simulink model "two_level_seriesparallel_spwm"  (R2016a)
settings: Solver=VariableStepAuto  StartTime=0.0  StopTime=stop_time  RelTol=1e-3
values from neighbouring files (symbols this model uses):
  DC_Voltage_Source = 540    [spectrumanalysis.m]
  DCLINK1_Cap = 100e-6    (= 0.0001)    [spectrumanalysis.m]
  DCLINK2_Cap = 100e-6    (= 0.0001)    [spectrumanalysis.m]
  interleaving_angle = 180    [spectrumanalysis.m]
  Load_Inductive_Power = 4116    [spectrumanalysis.m]
  Load_Real_Power = 8500    [spectrumanalysis.m]
  ma = 1    [spectrumanalysis.m]
  ref_frequency = 2*pi*50    (= 314.159265359)    [spectrumanalysis.m]
  Sampling_time = 1/(20*sw_frequency)    (= 2.43902439024e-05)    [spectrumanalysis.m]
libraries: powerlib x65, powerlib_meascontrol x12, simulink x12
settings Model: Creator=hakan  LastModifiedBy=hakan
settings DataIOCC: LimitDataPoints=on
settings DebuggingCC: MaxConsecutiveZCsMsg=none  AllowSymbolicDim=off
settings ModelReferenceCC: PropagateSignalLabelsOutOfModel=off
settings GRTTargetCC: GeneratePreprocessorConditionals=Use local settings

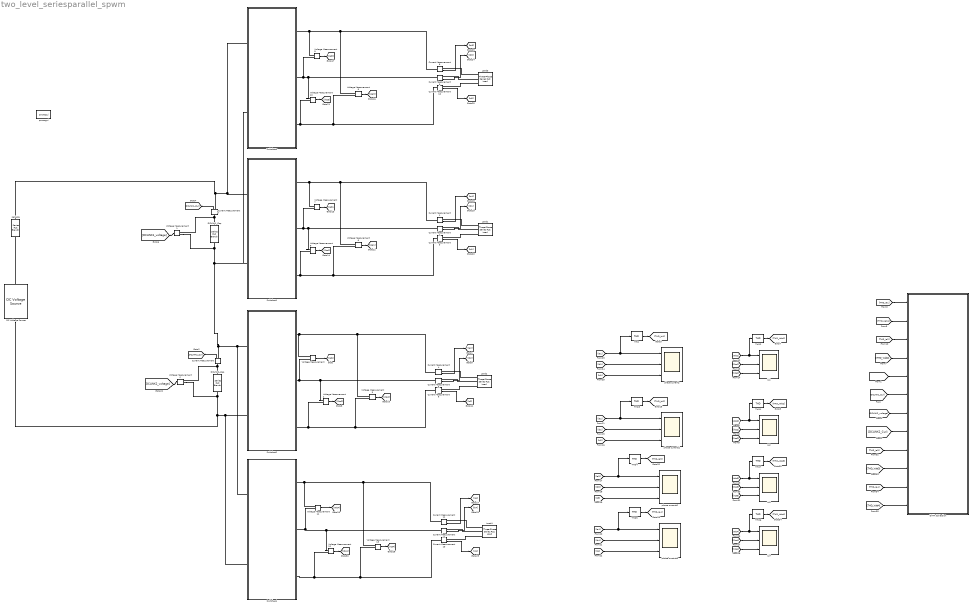
== system two_level_seriesparallel_spwm ==
  Current Measurement{,1..13} (14 alike) : powerlib/Measurements/Current Measurement  PhasorSimulation=off  OutputType=Complex  PSBequivalent=0
  DATA Collection : Subsystem
  DC Voltage Source : powerlib/Electrical Sources/DC Voltage Source  Amplitude=DC_Voltage_Source  Measurements=None
  DCLINK1_Cap : powerlib/Elements/Series RLC Branch  LConnTagsString=__new0  RConnTagsString=__new0  BranchType=C  Resistance=1  Inductance=1e-3  SetiL0=off  InitialCurrent=0  Capacitance=DCLINK1_Cap  Setx0=off  InitialVoltage=0  Measurements=None
  DCLINK2_Cap : powerlib/Elements/Series RLC Branch  LConnTagsString=__new0  RConnTagsString=__new0  BranchType=C  Resistance=1  Inductance=1e-3  SetiL0=off  InitialCurrent=0  Capacitance=DCLINK2_Cap  Setx0=off  InitialVoltage=0  Measurements=None
  LL{1..4} (4 alike) : Scope  NumInputPorts=3
  Load{1..4} (4 alike) : powerlib/Elements/Three-Phase Series RLC Load  LConnTagsString=A|B|C  Configuration=Y (floating)  NominalVoltage=1000  Vabc=[1e3 1e3 1e3]  Vabcp=[1e3 1e3 1e3]  NominalFrequency=Load_Nominal_Freq  UnbalancedPower=off  ActivePower=Load_Real_Power/4  InductivePower=Load_Inductive_Power/4  CapacitivePower=0  Pabc=[10e3 9e3 11e3]  QLabc=[100 90 110]  QCabc=[100 90 110]  Pabcp=[10e3 9e3 11e3]  QLabcp=[100 90 110]  QCabcp=[100 90 110]  Measurements=None  LoadType=constant Z
  Switches1 : Subsystem
  Switches2 : Subsystem
  Switches3 : Subsystem
  Switches4 : Subsystem
  THD{,1..7} (8 alike) : powerlib_meascontrol/Measurements/THD  Freq=50  Ts=0
  Voltage Measurement{,1..13} (14 alike) : powerlib/Measurements/Voltage Measurement  PhasorSimulation=off  OutputType=Complex  PSBequivalent=0
  phase currents{,1..3} (4 alike) : Scope  NumInputPorts=3
  powergui : powerlib/powergui  Priority=1  SimulationMode=Discrete  SolverType=Tustin/Backward Euler (TBE)  SampleTime=Sampling_time  frequency=60  SPID=off  DisableSnubberDevices=off  DisableRonSwitches=off  DisableVfSwitches=off  SwTol=0  DisplayEquations=off  Interpol=off  ExternalGateDelay=off  methode=off  Ts=10  FunctionMessages=off  echomessages=off  HookPort=off  EnableUseOfTLC=off  x0status=blocks  frequencyindice=0  Pbase=100e6  ErrMax=1e-4  Iterations=50  UnitsV=kV  UnitsW=MW  buscounter=0  RestoreLinks=warning  ResistiveCurrentMeasurement=off  Frange=[0:2:500]  Ylog=off  Xlog=on  ShowGrid=off  save=off  variable=ZData  structure=Phase_currents  ZoomFFT=off  StartTime=0.1  cycles=5  DisplayStyle=1  fundamental=50  FreqAxis=off  MaxFrequency=2000  frequencyindicesteady=1  RmsSteady=1  display=off
  seriesre : powerlib/Elements/Series RLC Branch  RequirementInfo={'linktype_rmi_matlab' 'C:\Users\hakan\Downloads\figuringout.m' '@737069.1' 'true' 'C' '' } %GIDa_c1573da4_5ff5_49fa_8615_7e57ae13da62  LConnTagsString=__new0  RConnTagsString=__new0  BranchType=R  Resistance=1  Inductance=1e-3  SetiL0=off  InitialCurrent=0  Capacitance=100e-6  Setx0=off  InitialVoltage=0  Measurements=Branch voltage and current
  wires:
  Current Measurement1/1 -> [Ia1]
  Current Measurement2/1 -> [Ib1]
  Current Measurement3/1 -> [Ic1]
  [Ib1] -> phase currents/2  "Ib"
  [Ia1] -> phase currents/1, THD/1  "Ia"
  [Ic1] -> phase currents/3  "Ic"
  [Vab1] -> THD2/1, LL1/1
  [Vbc1] -> LL1/2
  [Vca1] -> LL1/3
  THD/1 -> [THD_Ia1]
  [THD_Ia1] -> DATA Collection/1("THD_Ia1 ")
  THD2/1 -> [THD_Vab1]
  [THD_Vab2] -> DATA Collection/4(THD_Vab2)
  [THD_Vab1] -> DATA Collection/2(THD_Vab1)
  [DCLINK1_voltage] -> DATA Collection/5(DCLINK1_Voltage)
  [DCLINK1_Cur] -> DATA Collection/6(DCLINK1_Current)
  Current Measurement4/1 -> [Ia2]
  Current Measurement5/1 -> [Ib2]
  Current Measurement6/1 -> [Ic2]
  Voltage Measurement4/1 -> [DCLINK2_voltage]
  Current Measurement/1 -> [DCLINK2_Cur]
  Voltage Measurement1/1 -> [DCLINK1_voltage]
  Current Measurement7/1 -> [DCLINK1_Cur]
  [DCLINK2_voltage] -> DATA Collection/7(DCLINK2_Voltage)
  [DCLINK2_Cur] -> DATA Collection/8(DCLINK2_Current)
  Voltage Measurement/1 -> [Vab2]
  Voltage Measurement2/1 -> [Vbc2]
  Voltage Measurement3/1 -> [Vca2]
  Voltage Measurement6/1 -> [Vca1]
  Voltage Measurement7/1 -> [Vab1]
  Voltage Measurement8/1 -> [Vbc1]
  [Vab2] -> LL2/1, THD1/1
  [Vbc2] -> LL2/2
  [Vca2] -> LL2/3
  THD1/1 -> [THD_Vab2]
  [THD_Ia2] -> DATA Collection/3(THD_Ia2)
  [Ib2] -> phase currents1/2  "Ib"
  [Ia2] -> THD3/1, phase currents1/1  "Ia"
  [Ic2] -> phase currents1/3  "Ic"
  THD3/1 -> [THD_Ia2]
  Current Measurement8/1 -> [Ia3]
  Current Measurement9/1 -> [Ib3]
  Current Measurement10/1 -> [Ic3]
  Voltage Measurement5/1 -> [Vca3]
  Voltage Measurement9/1 -> [Vab3]
  Voltage Measurement10/1 -> [Vbc3]
  Current Measurement11/1 -> [Ia4]
  Current Measurement12/1 -> [Ib4]
  Current Measurement13/1 -> [Ic4]
  Voltage Measurement11/1 -> [Vab4]
  Voltage Measurement12/1 -> [Vbc4]
  Voltage Measurement13/1 -> [Vca4]
  [Ib3] -> phase currents2/2  "Ib"
  [Ia3] -> phase currents2/1, THD4/1  "Ia"
  [Ic3] -> phase currents2/3  "Ic"
  THD4/1 -> [THD_Ia3]
  [Ib4] -> phase currents3/2  "Ib"
  [Ia4] -> THD5/1, phase currents3/1  "Ia"
  [Ic4] -> phase currents3/3  "Ic"
  THD5/1 -> [THD_Ia4]
  [Vab4] -> THD6/1, LL4/1
  [Vbc4] -> LL4/2
  [Vca4] -> LL4/3
  THD6/1 -> [THD_Vab4]
  [Vab3] -> THD7/1, LL3/1
  [Vbc3] -> LL3/2
  [Vca3] -> LL3/3
  THD7/1 -> [THD_Vab3]
  [THD_Ia3] -> DATA Collection/9(THD_Ia3)
  [THD_Vab3] -> DATA Collection/10(THD_Vab3)
  [THD_Ia4] -> DATA Collection/11(THD_Ia4)
  [THD_Vab4] -> DATA Collection/12(THD_Vab4)
  connections:
  Load1/LConn1 -- Current Measurement1/RConn1
  Load1/LConn3 -- Current Measurement3/RConn1
  Load1/LConn2 -- Current Measurement2/RConn1
  Current Measurement1/LConn1 -- Voltage Measurement6/LConn2 -- Voltage Measurement7/LConn1 -- Switches1/RConn1
  Current Measurement2/LConn1 -- Voltage Measurement8/LConn1 -- Voltage Measurement7/LConn2 -- Switches1/RConn2
  Current Measurement3/LConn1 -- Voltage Measurement6/LConn1 -- Voltage Measurement8/LConn2 -- Switches1/RConn3
  Load2/LConn2 -- Current Measurement5/RConn1
  Load2/LConn3 -- Current Measurement6/RConn1
  Load2/LConn1 -- Current Measurement4/RConn1
  Current Measurement5/LConn1 -- Voltage Measurement2/LConn1 -- Voltage Measurement/LConn2 -- Switches2/RConn2
  Current Measurement4/LConn1 -- Voltage Measurement3/LConn2 -- Voltage Measurement/LConn1 -- Switches2/RConn1
  Current Measurement6/LConn1 -- Voltage Measurement3/LConn1 -- Voltage Measurement2/LConn2 -- Switches2/RConn3
  Voltage Measurement1/LConn2 -- Switches3/LConn2 -- Switches1/LConn2 -- Current Measurement/RConn1 -- Switches4/LConn1 -- Switches2/LConn1 -- DCLINK1_Cap/RConn1
  DC Voltage Source/LConn1 -- Voltage Measurement4/LConn2 -- DCLINK2_Cap/RConn1 -- Switches4/LConn2 -- Switches2/LConn2
  DC Voltage Source/RConn1 -- seriesre/RConn1
  seriesre/LConn1 -- Current Measurement7/RConn1 -- Switches3/LConn1 -- Switches1/LConn1
  DCLINK2_Cap/LConn1 -- Current Measurement/LConn1 -- Voltage Measurement4/LConn1
  DCLINK1_Cap/LConn1 -- Voltage Measurement1/LConn1 -- Current Measurement7/LConn1
  Current Measurement8/LConn1 -- Switches3/RConn1 -- Voltage Measurement9/LConn1 -- Voltage Measurement5/LConn2
  Current Measurement9/LConn1 -- Switches3/RConn2 -- Voltage Measurement9/LConn2 -- Voltage Measurement10/LConn1
  Current Measurement10/LConn1 -- Switches3/RConn3 -- Voltage Measurement10/LConn2 -- Voltage Measurement5/LConn1
  Load3/LConn3 -- Current Measurement10/RConn1
  Load3/LConn1 -- Current Measurement8/RConn1
  Load3/LConn2 -- Current Measurement9/RConn1
  Current Measurement12/LConn1 -- Voltage Measurement11/LConn2 -- Switches4/RConn2 -- Voltage Measurement12/LConn1
  Current Measurement11/LConn1 -- Voltage Measurement13/LConn2 -- Voltage Measurement11/LConn1 -- Switches4/RConn1
  Current Measurement13/LConn1 -- Voltage Measurement12/LConn2 -- Switches4/RConn3 -- Voltage Measurement13/LConn1
  Load4/LConn2 -- Current Measurement12/RConn1
  Load4/LConn1 -- Current Measurement11/RConn1
  Load4/LConn3 -- Current Measurement13/RConn1

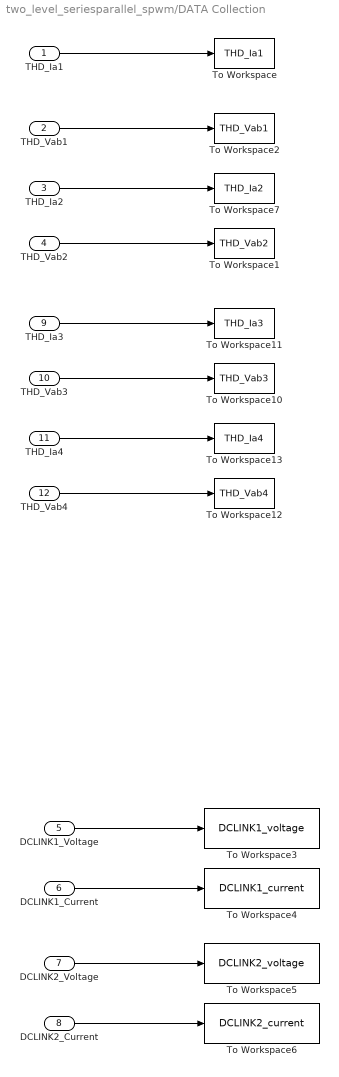
== system two_level_seriesparallel_spwm/DATA Collection ==
  "THD_Ia1 " : Inport
  THD_Vab1 : Inport  Port=2
  THD_Ia2 : Inport  Port=3
  THD_Vab2 : Inport  Port=4
  DCLINK1_Voltage : Inport  Port=5
  DCLINK1_Current : Inport  Port=6
  DCLINK2_Voltage : Inport  Port=7
  DCLINK2_Current : Inport  Port=8
  THD_Ia3 : Inport  Port=9
  THD_Vab3 : Inport  Port=10
  THD_Ia4 : Inport  Port=11
  THD_Vab4 : Inport  Port=12
  To Workspace : ToWorkspace  VariableName=THD_Ia1  SaveFormat=Timeseries  SampleTime=-1
  To Workspace1 : ToWorkspace  VariableName=THD_Vab2  SaveFormat=Timeseries  SampleTime=-1
  To Workspace10 : ToWorkspace  VariableName=THD_Vab3  SaveFormat=Timeseries  SampleTime=-1
  To Workspace11 : ToWorkspace  VariableName=THD_Ia3  SaveFormat=Timeseries  SampleTime=-1
  To Workspace12 : ToWorkspace  VariableName=THD_Vab4  SaveFormat=Timeseries  SampleTime=-1
  To Workspace13 : ToWorkspace  VariableName=THD_Ia4  SaveFormat=Timeseries  SampleTime=-1
  To Workspace2 : ToWorkspace  VariableName=THD_Vab1  SaveFormat=Timeseries  SampleTime=-1
  To Workspace3 : ToWorkspace  VariableName=DCLINK1_voltage  SaveFormat=Timeseries  SampleTime=-1
  To Workspace4 : ToWorkspace  VariableName=DCLINK1_current  SaveFormat=Timeseries  SampleTime=-1
  To Workspace5 : ToWorkspace  VariableName=DCLINK2_voltage  SaveFormat=Timeseries  SampleTime=-1
  To Workspace6 : ToWorkspace  VariableName=DCLINK2_current  SaveFormat=Timeseries  SampleTime=-1
  To Workspace7 : ToWorkspace  VariableName=THD_Ia2  SaveFormat=Timeseries  SampleTime=-1
  wires:
  DCLINK1_Voltage/1 -> To Workspace3/1
  THD_Vab1/1 -> To Workspace2/1
  "THD_Ia1 "/1 -> To Workspace/1
  THD_Vab2/1 -> To Workspace1/1
  DCLINK1_Current/1 -> To Workspace4/1
  DCLINK2_Voltage/1 -> To Workspace5/1
  DCLINK2_Current/1 -> To Workspace6/1
  THD_Ia2/1 -> To Workspace7/1
  THD_Vab3/1 -> To Workspace10/1
  THD_Ia3/1 -> To Workspace11/1
  THD_Ia4/1 -> To Workspace13/1
  THD_Vab4/1 -> To Workspace12/1

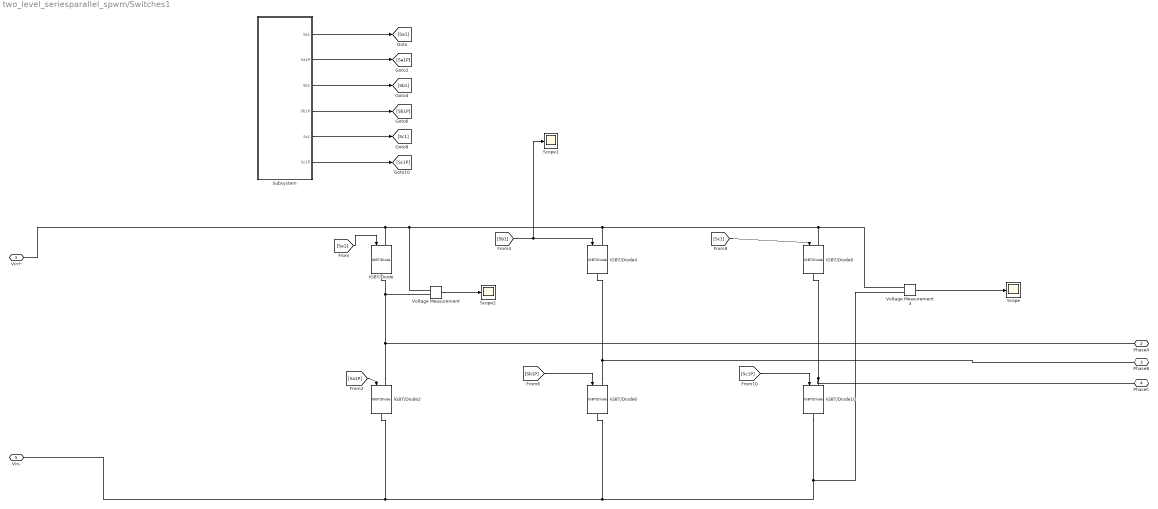
== system two_level_seriesparallel_spwm/Switches1 ==
  IGBT/Diode{,2,4,6,8,10} (6 alike) : powerlib/Power Electronics/IGBT//Diode  Ron=1e-3  Rs=1e5  Cs=inf  Measurements=off
  Scope : Scope
  Scope1 : Scope
  Scope2 : Scope
  Subsystem : Subsystem
  Voltage Measurement : powerlib/Measurements/Voltage Measurement  PhasorSimulation=off  OutputType=Complex  PSBequivalent=0
  Voltage Measurement3 : powerlib/Measurements/Voltage Measurement  PhasorSimulation=off  OutputType=Complex  PSBequivalent=0
  Vin+ : PMIOPort  Port=1  Side=Left
  PhaseA : PMIOPort  Port=2  Side=Right
  PhaseB : PMIOPort  Port=3  Side=Right
  PhaseC : PMIOPort  Port=4  Side=Right
  Vin- : PMIOPort  Port=5  Side=Left
  wires:
  [Sc1P] -> IGBT/Diode10/1
  [Sb1P] -> IGBT/Diode6/1
  [Sa1] -> IGBT/Diode/1
  [Sb1] -> Scope1/1, IGBT/Diode4/1
  [Sa1P] -> IGBT/Diode2/1
  [Sc1] -> IGBT/Diode8/1
  Voltage Measurement3/1 -> Scope/1
  Subsystem/1("Sa1 ") -> [Sa1]
  Subsystem/2(Sa1P) -> [Sa1P]
  Subsystem/3(Sb1) -> [Sb1]
  Subsystem/6(Sc1P) -> [Sc1P]
  Subsystem/5(Sc1) -> [Sc1]
  Subsystem/4(Sb1P) -> [Sb1P]
  Voltage Measurement/1 -> Scope2/1
  connections:
  IGBT/Diode2/LConn1 -- PhaseA/RConn1 -- Voltage Measurement/LConn2 -- IGBT/Diode/RConn1
  IGBT/Diode6/RConn1 -- Voltage Measurement3/LConn2 -- IGBT/Diode10/RConn1 -- Vin-/RConn1 -- IGBT/Diode2/RConn1
  IGBT/Diode8/RConn1 -- PhaseC/RConn1 -- IGBT/Diode10/LConn1
  IGBT/Diode6/LConn1 -- PhaseB/RConn1 -- IGBT/Diode4/RConn1
  IGBT/Diode/LConn1 -- Voltage Measurement/LConn1 -- Voltage Measurement3/LConn1 -- IGBT/Diode8/LConn1 -- IGBT/Diode4/LConn1 -- Vin+/RConn1

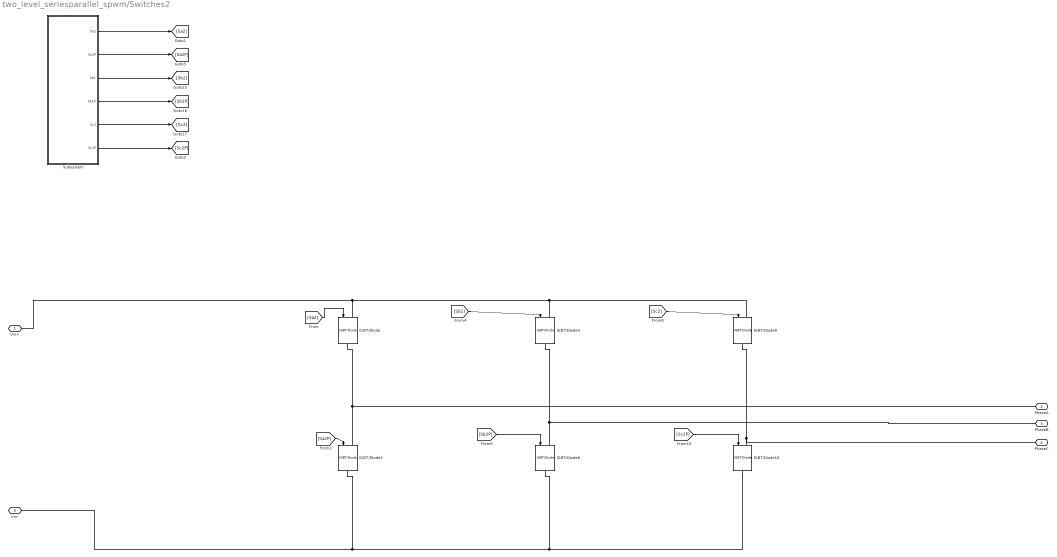
== system two_level_seriesparallel_spwm/Switches2 ==
  IGBT/Diode{,2,4,6,8,10} (6 alike) : powerlib/Power Electronics/IGBT//Diode  Ron=1e-3  Rs=1e5  Cs=inf  Measurements=off
  Subsystem : Subsystem
  Vin+ : PMIOPort  Port=1  Side=Left
  PhaseA : PMIOPort  Port=2  Side=Right
  PhaseB : PMIOPort  Port=3  Side=Right
  PhaseC : PMIOPort  Port=4  Side=Right
  Vin- : PMIOPort  Port=5  Side=Left
  wires:
  [Sc2] -> IGBT/Diode8/1
  [Sa2P] -> IGBT/Diode2/1
  [Sb2] -> IGBT/Diode4/1
  [Sa2] -> IGBT/Diode/1
  [Sb2P] -> IGBT/Diode6/1
  [Sc2P] -> IGBT/Diode10/1
  Subsystem/1("Sa1 ") -> [Sa2]
  Subsystem/2(Sa1P) -> [Sa2P]
  Subsystem/3(Sb1) -> [Sb2]
  Subsystem/6(Sc1P) -> [Sc2P]
  Subsystem/5(Sc1) -> [Sc2]
  Subsystem/4(Sb1P) -> [Sb2P]
  connections:
  PhaseB/RConn1 -- IGBT/Diode6/LConn1 -- IGBT/Diode4/RConn1
  PhaseC/RConn1 -- IGBT/Diode8/RConn1 -- IGBT/Diode10/LConn1
  Vin+/RConn1 -- IGBT/Diode/LConn1 -- IGBT/Diode8/LConn1 -- IGBT/Diode4/LConn1
  PhaseA/RConn1 -- IGBT/Diode/RConn1 -- IGBT/Diode2/LConn1
  Vin-/RConn1 -- IGBT/Diode6/RConn1 -- IGBT/Diode10/RConn1 -- IGBT/Diode2/RConn1

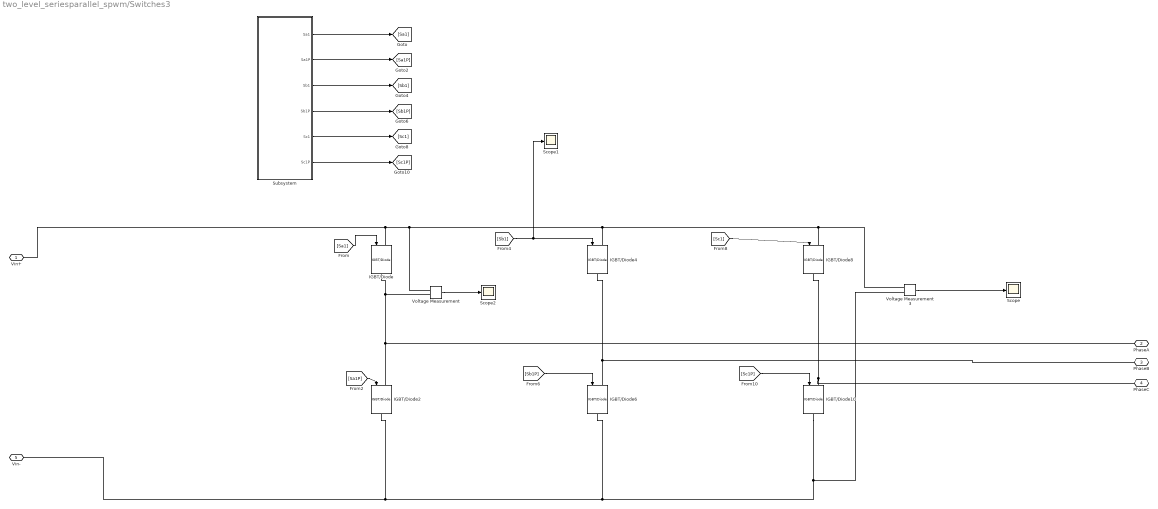
== system two_level_seriesparallel_spwm/Switches3 ==
  IGBT/Diode{,2,4,6,8,10} (6 alike) : powerlib/Power Electronics/IGBT//Diode  Ron=1e-3  Rs=1e5  Cs=inf  Measurements=off
  Scope : Scope
  Scope1 : Scope
  Scope2 : Scope
  Subsystem : Subsystem
  Voltage Measurement : powerlib/Measurements/Voltage Measurement  PhasorSimulation=off  OutputType=Complex  PSBequivalent=0
  Voltage Measurement3 : powerlib/Measurements/Voltage Measurement  PhasorSimulation=off  OutputType=Complex  PSBequivalent=0
  Vin+ : PMIOPort  Port=1  Side=Left
  PhaseA : PMIOPort  Port=2  Side=Right
  PhaseB : PMIOPort  Port=3  Side=Right
  PhaseC : PMIOPort  Port=4  Side=Right
  Vin- : PMIOPort  Port=5  Side=Left
  wires:
  Voltage Measurement/1 -> Scope2/1
  Subsystem/4(Sb1P) -> [Sb1P]
  Subsystem/5(Sc1) -> [Sc1]
  Subsystem/6(Sc1P) -> [Sc1P]
  Subsystem/3(Sb1) -> [Sb1]
  Subsystem/2(Sa1P) -> [Sa1P]
  Subsystem/1("Sa1 ") -> [Sa1]
  Voltage Measurement3/1 -> Scope/1
  [Sc1] -> IGBT/Diode8/1
  [Sa1P] -> IGBT/Diode2/1
  [Sb1] -> IGBT/Diode4/1, Scope1/1
  [Sa1] -> IGBT/Diode/1
  [Sb1P] -> IGBT/Diode6/1
  [Sc1P] -> IGBT/Diode10/1
  connections:
  Vin+/RConn1 -- IGBT/Diode4/LConn1 -- IGBT/Diode8/LConn1 -- Voltage Measurement3/LConn1 -- Voltage Measurement/LConn1 -- IGBT/Diode/LConn1
  IGBT/Diode4/RConn1 -- PhaseB/RConn1 -- IGBT/Diode6/LConn1
  IGBT/Diode10/LConn1 -- PhaseC/RConn1 -- IGBT/Diode8/RConn1
  IGBT/Diode2/RConn1 -- Vin-/RConn1 -- IGBT/Diode10/RConn1 -- Voltage Measurement3/LConn2 -- IGBT/Diode6/RConn1
  IGBT/Diode/RConn1 -- Voltage Measurement/LConn2 -- PhaseA/RConn1 -- IGBT/Diode2/LConn1

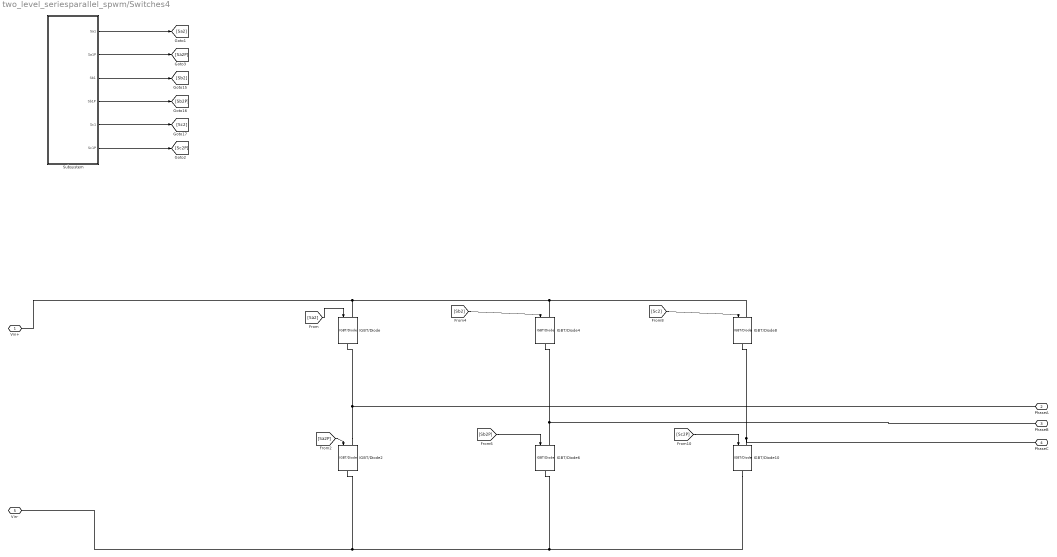
== system two_level_seriesparallel_spwm/Switches4 ==
  IGBT/Diode{,2,4,6,8,10} (6 alike) : powerlib/Power Electronics/IGBT//Diode  Ron=1e-3  Rs=1e5  Cs=inf  Measurements=off
  Subsystem : Subsystem
  Vin+ : PMIOPort  Port=1  Side=Left
  PhaseA : PMIOPort  Port=2  Side=Right
  PhaseB : PMIOPort  Port=3  Side=Right
  PhaseC : PMIOPort  Port=4  Side=Right
  Vin- : PMIOPort  Port=5  Side=Left
  wires:
  Subsystem/4(Sb1P) -> [Sb2P]
  Subsystem/5(Sc1) -> [Sc2]
  Subsystem/6(Sc1P) -> [Sc2P]
  Subsystem/3(Sb1) -> [Sb2]
  Subsystem/2(Sa1P) -> [Sa2P]
  Subsystem/1("Sa1 ") -> [Sa2]
  [Sc2P] -> IGBT/Diode10/1
  [Sb2P] -> IGBT/Diode6/1
  [Sa2] -> IGBT/Diode/1
  [Sb2] -> IGBT/Diode4/1
  [Sa2P] -> IGBT/Diode2/1
  [Sc2] -> IGBT/Diode8/1
  connections:
  IGBT/Diode2/RConn1 -- IGBT/Diode10/RConn1 -- IGBT/Diode6/RConn1 -- Vin-/RConn1
  IGBT/Diode2/LConn1 -- IGBT/Diode/RConn1 -- PhaseA/RConn1
  IGBT/Diode4/LConn1 -- IGBT/Diode8/LConn1 -- IGBT/Diode/LConn1 -- Vin+/RConn1
  IGBT/Diode10/LConn1 -- IGBT/Diode8/RConn1 -- PhaseC/RConn1
  IGBT/Diode4/RConn1 -- IGBT/Diode6/LConn1 -- PhaseB/RConn1

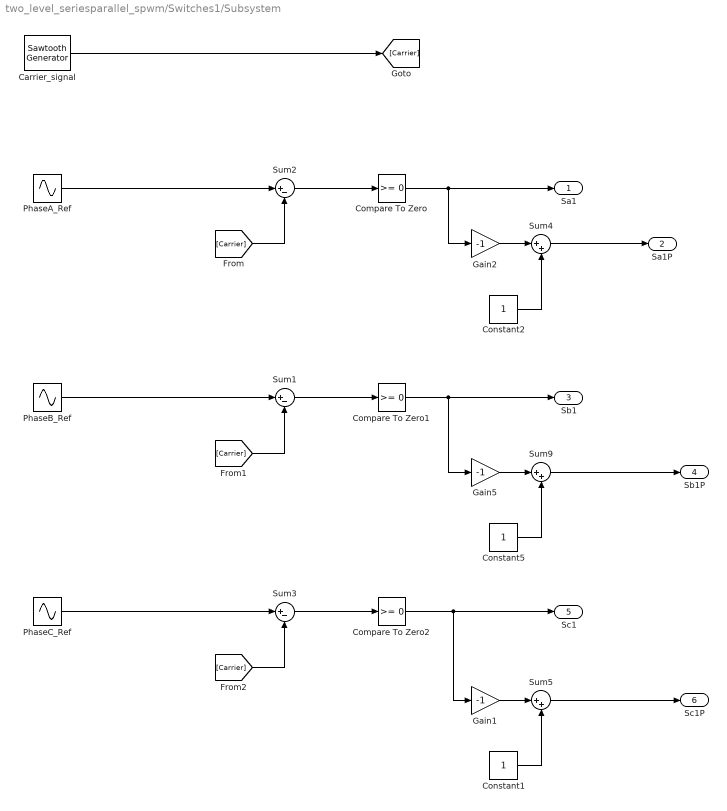
== system two_level_seriesparallel_spwm/Switches1/Subsystem ==
  Carrier_signal : powerlib_meascontrol/Pulse & Signal Generators/Sawtooth Generator  Freq=sw_frequency  Phase=0  Ts=0
  Compare To Zero : simulink/Logic and Bit Operations/Compare To Zero  relop=>=  OutDataTypeStr=boolean
  Compare To Zero1 : simulink/Logic and Bit Operations/Compare To Zero  relop=>=  OutDataTypeStr=boolean
  Compare To Zero2 : simulink/Logic and Bit Operations/Compare To Zero  relop=>=  OutDataTypeStr=boolean
  Constant1 : Constant
  Constant2 : Constant
  Constant5 : Constant
  Gain1 : Gain  Gain=-1
  Gain2 : Gain  Gain=-1
  Gain5 : Gain  Gain=-1
  PhaseA_Ref : Sin  Amplitude=ma  Frequency=ref_frequency  SampleTime=0
  PhaseB_Ref : Sin  Amplitude=ma  Frequency=ref_frequency  Phase=2*pi/3  SampleTime=0
  PhaseC_Ref : Sin  Amplitude=ma  Frequency=ref_frequency  Phase=4*pi/3  SampleTime=0
  Sum1 : Sum  Inputs=|+-
  Sum2 : Sum  Inputs=|+-
  Sum3 : Sum  Inputs=|+-
  Sum4 : Sum  Inputs=|++
  Sum5 : Sum  Inputs=|++
  Sum9 : Sum  Inputs=|++
  "Sa1 " : Outport
  Sa1P : Outport  Port=2
  Sb1 : Outport  Port=3
  Sb1P : Outport  Port=4
  Sc1 : Outport  Port=5
  Sc1P : Outport  Port=6
  wires:
  PhaseA_Ref/1 -> Sum2/1
  Sum4/1 -> Sa1P/1
  Gain2/1 -> Sum4/1
  Constant2/1 -> Sum4/2
  Compare To Zero/1 -> "Sa1 "/1, Gain2/1
  Sum2/1 -> Compare To Zero/1
  [Carrier] -> Sum2/2
  Carrier_signal/1 -> [Carrier]
  Compare To Zero1/1 -> Gain5/1, Sb1/1
  PhaseB_Ref/1 -> Sum1/1
  [Carrier] -> Sum1/2
  Compare To Zero2/1 -> Gain1/1, Sc1/1
  PhaseC_Ref/1 -> Sum3/1
  [Carrier] -> Sum3/2
  Sum1/1 -> Compare To Zero1/1
  Gain5/1 -> Sum9/1
  Sum9/1 -> Sb1P/1
  Constant5/1 -> Sum9/2
  Constant1/1 -> Sum5/2
  Sum5/1 -> Sc1P/1
  Sum3/1 -> Compare To Zero2/1
  Gain1/1 -> Sum5/1

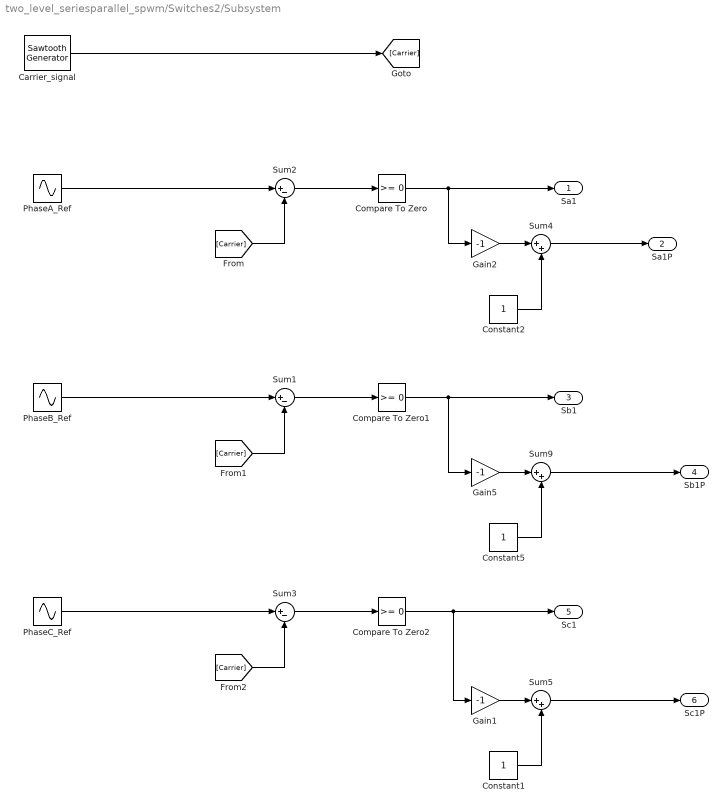
== system two_level_seriesparallel_spwm/Switches2/Subsystem ==
  Carrier_signal : powerlib_meascontrol/Pulse & Signal Generators/Sawtooth Generator  Freq=sw_frequency  Phase=0  Ts=0
  Compare To Zero : simulink/Logic and Bit Operations/Compare To Zero  relop=>=  OutDataTypeStr=boolean
  Compare To Zero1 : simulink/Logic and Bit Operations/Compare To Zero  relop=>=  OutDataTypeStr=boolean
  Compare To Zero2 : simulink/Logic and Bit Operations/Compare To Zero  relop=>=  OutDataTypeStr=boolean
  Constant1 : Constant
  Constant2 : Constant
  Constant5 : Constant
  Gain1 : Gain  Gain=-1
  Gain2 : Gain  Gain=-1
  Gain5 : Gain  Gain=-1
  PhaseA_Ref : Sin  Amplitude=ma  Frequency=ref_frequency  SampleTime=0
  PhaseB_Ref : Sin  Amplitude=ma  Frequency=ref_frequency  Phase=2*pi/3  SampleTime=0
  PhaseC_Ref : Sin  Amplitude=ma  Frequency=ref_frequency  Phase=4*pi/3  SampleTime=0
  Sum1 : Sum  Inputs=|+-
  Sum2 : Sum  Inputs=|+-
  Sum3 : Sum  Inputs=|+-
  Sum4 : Sum  Inputs=|++
  Sum5 : Sum  Inputs=|++
  Sum9 : Sum  Inputs=|++
  "Sa1 " : Outport
  Sa1P : Outport  Port=2
  Sb1 : Outport  Port=3
  Sb1P : Outport  Port=4
  Sc1 : Outport  Port=5
  Sc1P : Outport  Port=6
  wires:
  Gain1/1 -> Sum5/1
  Sum3/1 -> Compare To Zero2/1
  Sum5/1 -> Sc1P/1
  Constant1/1 -> Sum5/2
  Constant5/1 -> Sum9/2
  Sum9/1 -> Sb1P/1
  Gain5/1 -> Sum9/1
  Sum1/1 -> Compare To Zero1/1
  [Carrier] -> Sum3/2
  PhaseC_Ref/1 -> Sum3/1
  Compare To Zero2/1 -> Sc1/1, Gain1/1
  [Carrier] -> Sum1/2
  PhaseB_Ref/1 -> Sum1/1
  Compare To Zero1/1 -> Sb1/1, Gain5/1
  Carrier_signal/1 -> [Carrier]
  [Carrier] -> Sum2/2
  Sum2/1 -> Compare To Zero/1
  Compare To Zero/1 -> Gain2/1, "Sa1 "/1
  Constant2/1 -> Sum4/2
  Gain2/1 -> Sum4/1
  Sum4/1 -> Sa1P/1
  PhaseA_Ref/1 -> Sum2/1

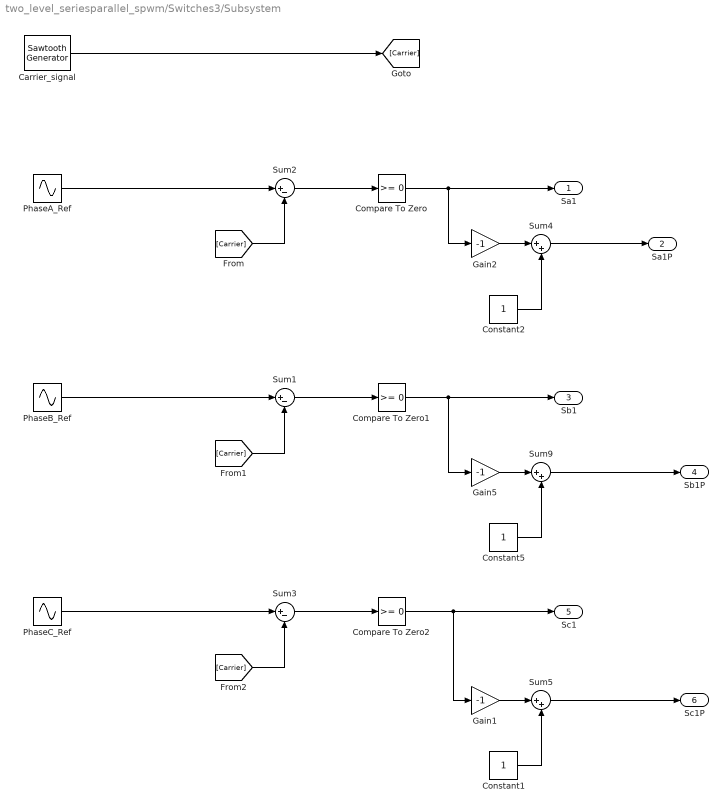
== system two_level_seriesparallel_spwm/Switches3/Subsystem ==
  Carrier_signal : powerlib_meascontrol/Pulse & Signal Generators/Sawtooth Generator  Freq=sw_frequency  Phase=interleaving_angle  Ts=0
  Compare To Zero : simulink/Logic and Bit Operations/Compare To Zero  relop=>=  OutDataTypeStr=boolean
  Compare To Zero1 : simulink/Logic and Bit Operations/Compare To Zero  relop=>=  OutDataTypeStr=boolean
  Compare To Zero2 : simulink/Logic and Bit Operations/Compare To Zero  relop=>=  OutDataTypeStr=boolean
  Constant1 : Constant
  Constant2 : Constant
  Constant5 : Constant
  Gain1 : Gain  Gain=-1
  Gain2 : Gain  Gain=-1
  Gain5 : Gain  Gain=-1
  PhaseA_Ref : Sin  Amplitude=ma  Frequency=ref_frequency  SampleTime=0
  PhaseB_Ref : Sin  Amplitude=ma  Frequency=ref_frequency  Phase=2*pi/3  SampleTime=0
  PhaseC_Ref : Sin  Amplitude=ma  Frequency=ref_frequency  Phase=4*pi/3  SampleTime=0
  Sum1 : Sum  Inputs=|+-
  Sum2 : Sum  Inputs=|+-
  Sum3 : Sum  Inputs=|+-
  Sum4 : Sum  Inputs=|++
  Sum5 : Sum  Inputs=|++
  Sum9 : Sum  Inputs=|++
  "Sa1 " : Outport
  Sa1P : Outport  Port=2
  Sb1 : Outport  Port=3
  Sb1P : Outport  Port=4
  Sc1 : Outport  Port=5
  Sc1P : Outport  Port=6
  wires:
  Gain1/1 -> Sum5/1
  Sum3/1 -> Compare To Zero2/1
  Sum5/1 -> Sc1P/1
  Constant1/1 -> Sum5/2
  Constant5/1 -> Sum9/2
  Sum9/1 -> Sb1P/1
  Gain5/1 -> Sum9/1
  Sum1/1 -> Compare To Zero1/1
  [Carrier] -> Sum3/2
  PhaseC_Ref/1 -> Sum3/1
  Compare To Zero2/1 -> Sc1/1, Gain1/1
  [Carrier] -> Sum1/2
  PhaseB_Ref/1 -> Sum1/1
  Compare To Zero1/1 -> Sb1/1, Gain5/1
  Carrier_signal/1 -> [Carrier]
  [Carrier] -> Sum2/2
  Sum2/1 -> Compare To Zero/1
  Compare To Zero/1 -> Gain2/1, "Sa1 "/1
  Constant2/1 -> Sum4/2
  Gain2/1 -> Sum4/1
  Sum4/1 -> Sa1P/1
  PhaseA_Ref/1 -> Sum2/1

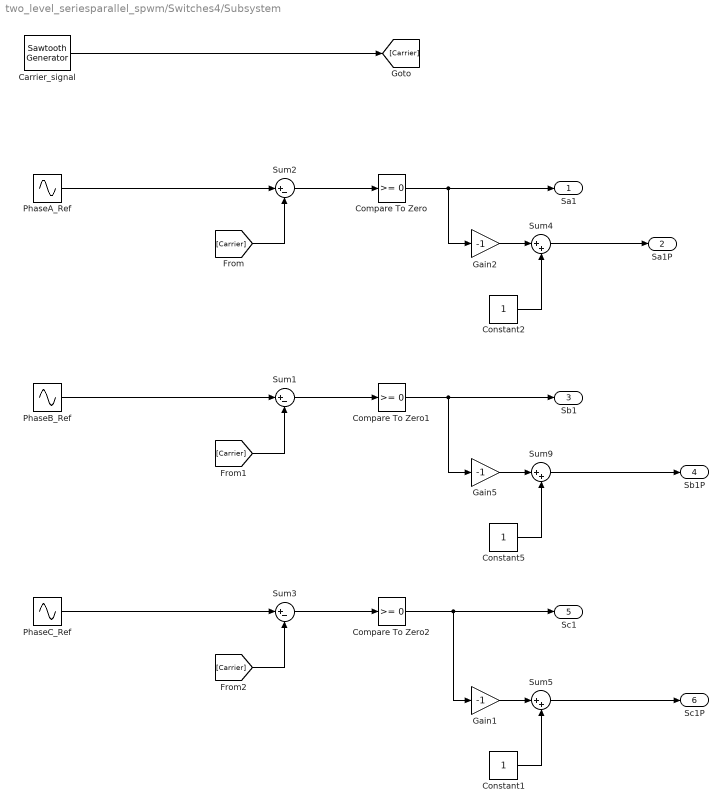
== system two_level_seriesparallel_spwm/Switches4/Subsystem ==
  Carrier_signal : powerlib_meascontrol/Pulse & Signal Generators/Sawtooth Generator  Freq=sw_frequency  Phase=interleaving_angle  Ts=0
  Compare To Zero : simulink/Logic and Bit Operations/Compare To Zero  relop=>=  OutDataTypeStr=boolean
  Compare To Zero1 : simulink/Logic and Bit Operations/Compare To Zero  relop=>=  OutDataTypeStr=boolean
  Compare To Zero2 : simulink/Logic and Bit Operations/Compare To Zero  relop=>=  OutDataTypeStr=boolean
  Constant1 : Constant
  Constant2 : Constant
  Constant5 : Constant
  Gain1 : Gain  Gain=-1
  Gain2 : Gain  Gain=-1
  Gain5 : Gain  Gain=-1
  PhaseA_Ref : Sin  Amplitude=ma  Frequency=ref_frequency  SampleTime=0
  PhaseB_Ref : Sin  Amplitude=ma  Frequency=ref_frequency  Phase=2*pi/3  SampleTime=0
  PhaseC_Ref : Sin  Amplitude=ma  Frequency=ref_frequency  Phase=4*pi/3  SampleTime=0
  Sum1 : Sum  Inputs=|+-
  Sum2 : Sum  Inputs=|+-
  Sum3 : Sum  Inputs=|+-
  Sum4 : Sum  Inputs=|++
  Sum5 : Sum  Inputs=|++
  Sum9 : Sum  Inputs=|++
  "Sa1 " : Outport
  Sa1P : Outport  Port=2
  Sb1 : Outport  Port=3
  Sb1P : Outport  Port=4
  Sc1 : Outport  Port=5
  Sc1P : Outport  Port=6
  wires:
  PhaseA_Ref/1 -> Sum2/1
  Sum4/1 -> Sa1P/1
  Gain2/1 -> Sum4/1
  Constant2/1 -> Sum4/2
  Compare To Zero/1 -> "Sa1 "/1, Gain2/1
  Sum2/1 -> Compare To Zero/1
  [Carrier] -> Sum2/2
  Carrier_signal/1 -> [Carrier]
  Compare To Zero1/1 -> Gain5/1, Sb1/1
  PhaseB_Ref/1 -> Sum1/1
  [Carrier] -> Sum1/2
  Compare To Zero2/1 -> Gain1/1, Sc1/1
  PhaseC_Ref/1 -> Sum3/1
  [Carrier] -> Sum3/2
  Sum1/1 -> Compare To Zero1/1
  Gain5/1 -> Sum9/1
  Sum9/1 -> Sb1P/1
  Constant5/1 -> Sum9/2
  Constant1/1 -> Sum5/2
  Sum5/1 -> Sc1P/1
  Sum3/1 -> Compare To Zero2/1
  Gain1/1 -> Sum5/1
